simulink model "lr24"  (R2021b)
settings: Solver=VariableStepAuto  StartTime=0.0  StopTime=10.0  RelTol=1e-3
values from neighbouring files (symbols this model uses):
  g = 9.81*m/s^2    (= 9.81)    [lr24_cruise.m]
  Iy = 18800*slug*ft^2    (= 25489.3722986)    [lr24_cruise.m]
  m = 13000*lb    (= 5896.70081)    [lr24_cruise.m]
  theta0 = alpha0    [lr24_cruise.m]
  u0 = tas*cos(alpha0)    [lr24_cruise.m]
  w0 = tas*sin(alpha0)    [lr24_cruise.m]
settings Model: Creator=cleme  LastModifiedBy=cleme

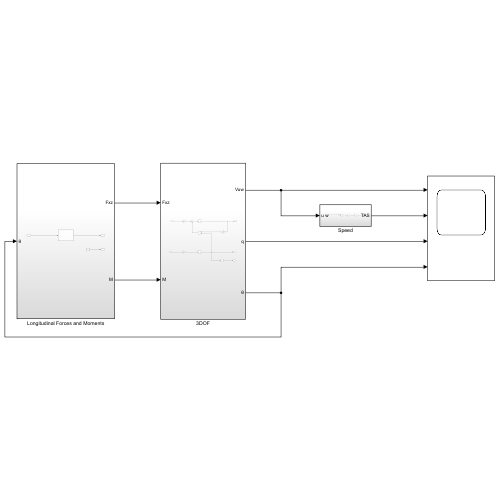
[thumbnail: Simulink's stored preview of the top-level diagram]
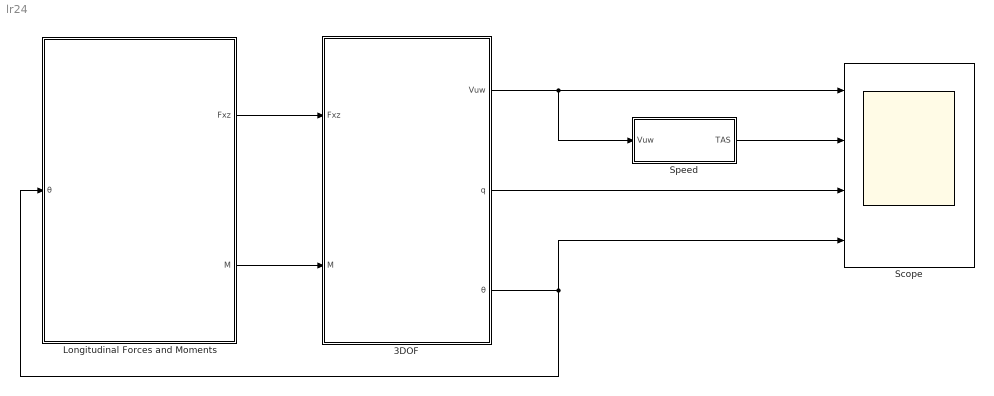
== system lr24 ==
  3DOF : Subsystem
  Longitudinal Forces and Moments : Subsystem
  Scope : Scope  NumInputPorts=4
  Speed : Subsystem
  wires:
  Longitudinal Forces and Moments/1(Fxz) -> 3DOF/1(Fxz)
  Longitudinal Forces and Moments/2(M) -> 3DOF/2(M)
  3DOF/3(θ) -> Longitudinal Forces and Moments/1(θ), Scope/4
  Speed/1(TAS) -> Scope/2
  3DOF/1(Vuw) -> Speed/1(Vuw), Scope/1
  3DOF/2(q) -> Scope/3

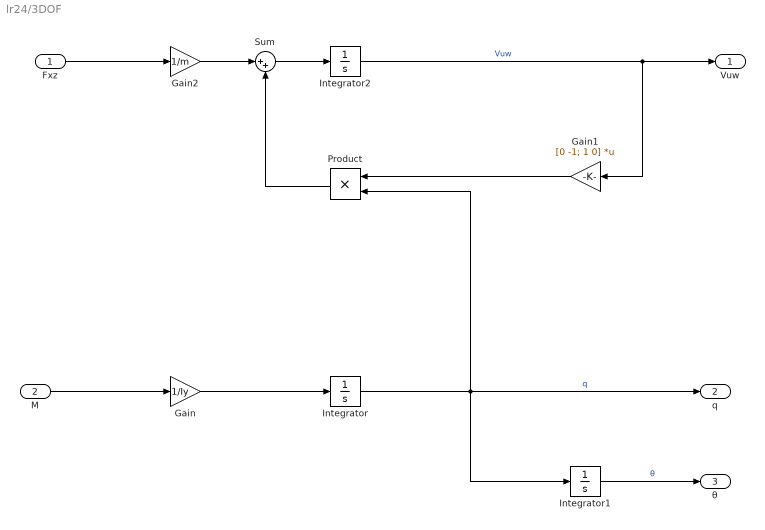
== system lr24/3DOF ==
  Fxz : Inport  Unit=N
  M : Inport  Port=2  Unit=N*m
  Gain : Gain  Gain=1/Iy
  Gain1 : Gain  Gain=[0 -1; 1 0]  Multiplication=Matrix(K*u)
      settings: AttributesFormatString=K = %<Gain>
  Gain2 : Gain  Gain=1/m
  Integrator : Integrator
  Integrator1 : Integrator  InitialCondition=theta0
  Integrator2 : Integrator  InitialCondition=[u0 w0]
  Product : Product
  Sum : Sum  Inputs=|++
  Vuw : Outport  Unit=m/s
  q : Outport  Port=2  Unit=rad/s
  θ : Outport  Port=3  Unit=rad
  wires:
  Integrator1/1 -> θ/1  "θ"
  M/1 -> Gain/1
  Gain/1 -> Integrator/1
  Integrator/1 -> Integrator1/1, Product/2, q/1  "q"
  Fxz/1 -> Gain2/1
  Gain2/1 -> Sum/1
  Integrator2/1 -> Gain1/1, Vuw/1  "Vuw"
  Gain1/1 -> Product/1
  Product/1 -> Sum/2
  Sum/1 -> Integrator2/1

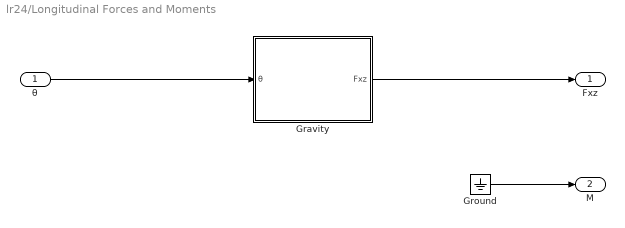
== system lr24/Longitudinal Forces and Moments ==
  θ : Inport
  Gravity : Subsystem
  Ground : Ground
  Fxz : Outport
  M : Outport  Port=2
  wires:
  Gravity/1(Fxz) -> Fxz/1
  Ground/1 -> M/1
  θ/1 -> Gravity/1(θ)

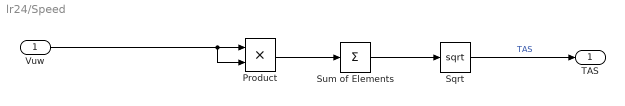
== system lr24/Speed ==
  Vuw : Inport
  Product : Product
  Sqrt : Sqrt  SaturateOnIntegerOverflow=on
  Sum of Elements : Sum  Inputs=+
  TAS : Outport
  wires:
  Vuw/1 -> Product/2, Product/1
  Product/1 -> Sum of Elements/1
  Sqrt/1 -> TAS/1  "TAS"
  Sum of Elements/1 -> Sqrt/1

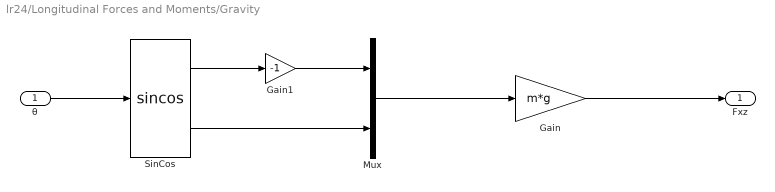
== system lr24/Longitudinal Forces and Moments/Gravity ==
  θ : Inport  Unit=rad
  Gain : Gain  Gain=m*g
  Gain1 : Gain  Gain=-1
  Mux : Mux  Inputs=2
  SinCos : Trigonometry  Operator=sincos
  Fxz : Outport
  wires:
  Gain/1 -> Fxz/1
  θ/1 -> SinCos/1
  SinCos/2 -> Mux/2
  Gain1/1 -> Mux/1
  Mux/1 -> Gain/1
  SinCos/1 -> Gain1/1
